simulink model "T3_updatesolarpart"  (R2022b)
settings: Solver=VariableStepAuto  StartTime=0.0  StopTime=10.0  RelTol=1e-3
undefined symbols (not defined in the file): High, Low
libraries: fl_lib x101, nesl_utility x52, simulink x14, ee_lib x5, slpidlib x2, eePwmGenerator x1
(part 3 of 3)

== system T3_updatesolarpart/Solar power/V ==
  PS-Simulink Converter : nesl_utility/PS-Simulink Converter  PhysicalDomain=network_engine_domain  SubClassName=ps_output  LeftPortType=input  RightPortType=output  PseudoPeriodic=off  Frequencies=[]  VectorFormat=inherit  Unit=inherit  AffineConversion=off
  Voltage Sensor : fl_lib/Electrical/Electrical Sensors/Voltage Sensor
  + : PMIOPort  Side=Left
  - : PMIOPort  Port=2  Side=Right
  tag scope: Vs=global
  wires:
  PS-Simulink Converter/1 -> [Vs]
  connections:
  PS-Simulink Converter/LConn1 -- Voltage Sensor/RConn1
  Voltage Sensor/LConn1 -- +/RConn1
  Voltage Sensor/RConn2 -- -/RConn1

== system T3_updatesolarpart/Wind energy/Subsystem ==
  Wind speed : Inport
  MATLAB System : MATLABSystem  System=windturbine_pitch_control  turbine_Pinst=1e6  turbine_dynamicsTimeConstant=5  inertia_dynamicsTimeConstant=3  Ts=0.01  SimulateUsing=Code generation
      mask Type: windturbine_pitch_control
      mask Display:
      | disp('windturbine_pitch_control');
      | port_label('input',1,'P_mechanic');
      | port_label('output',1,'P');
  Scope : Scope  NumInputPorts=2
  Wind turbine : Subsystem  mask{C1=0.5, C2=116, C3=0.4, C4=0, C5=5, C6=21, theta=0, W=1.57, R=40}
      mask prompts: C1 "coefficients C1"; C2 "coefficients C2"; C3 "coefficients C3"; C4 "coefficients C4"; C5 "coefficients C5"; C6 "coefficients C6"; theta "pitch angle"; W "angular velocity of rotor"; R "Blade Radius"
      mask DialogControl Container4 Prompt: Cp power coefficient
      mask DialogControl Container3 Prompt: Blade parameter
  Acitve power : Outport
  wires:
  Wind speed/1 -> Wind turbine/1(Vw wind speed)
  MATLAB System/1 -> Acitve power/1, Scope/2  "electrical"
  Wind turbine/1(Wind power) -> Scope/1, MATLAB System/1  "mechanical"

== system T3_updatesolarpart/Solar power/Boost Converter/AC Current Sensor1 ==
  Current Sensor : fl_lib/Electrical/Electrical Sensors/Current Sensor
  PS-Simulink Converter : nesl_utility/PS-Simulink Converter  PhysicalDomain=network_engine_domain  SubClassName=ps_output  LeftPortType=input  RightPortType=output  PseudoPeriodic=off  Frequencies=[]  VectorFormat=1-D array  Unit=1  AffineConversion=off
  - : PMIOPort  Side=Left
  + : PMIOPort  Port=2  Side=Right
  tag scope: Iboost=global
  wires:
  PS-Simulink Converter/1 -> [Iboost]
  connections:
  Current Sensor/RConn1 -- PS-Simulink Converter/LConn1
  +/RConn1 -- Current Sensor/LConn1
  Current Sensor/RConn2 -- -/RConn1

== system T3_updatesolarpart/Wind energy/Subsystem/Wind turbine ==
  Vw wind speed : Inport
  Blade radius : Constant  Value=R
  Constant : Constant  Value=1.225
  Multiply : Gain  Gain=1/2
  Multiply1 : Gain  Gain=pi
  Product : Product  Inputs=4
  Square : Math  Operator=square
  Subsystem : Subsystem
      mask Display: disp('Vw^3');
  Subsystem1 : Subsystem
  Wind power : Outport
  wires:
  Multiply/1 -> Wind power/1
  Product/1 -> Multiply/1
  Constant/1 -> Product/1  "Air density"
  Blade radius/1 -> Square/1
  Square/1 -> Multiply1/1
  Multiply1/1 -> Product/2  "Area"
  Vw wind speed/1 -> Subsystem1/1(Vw), Subsystem/1(In1)
  Subsystem1/1(Cp) -> Product/4
  Subsystem/1(Out1) -> Product/3

== system T3_updatesolarpart/Wind energy/Subsystem/Wind turbine/Subsystem ==
  In1 : Inport
  Square1 : Math  Operator=pow
  power of 3 : Constant  Value=3
  Out1 : Outport
  wires:
  power of 3/1 -> Square1/2
  Square1/1 -> Out1/1
  In1/1 -> Square1/1

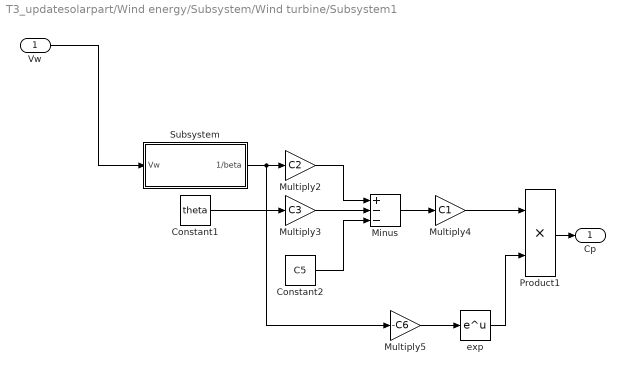
== system T3_updatesolarpart/Wind energy/Subsystem/Wind turbine/Subsystem1 ==
  Vw : Inport
  Constant1 : Constant  Value=theta
  Constant2 : Constant  Value=C5
  Minus : Sum  Inputs=+--
  Multiply2 : Gain  Gain=C2
  Multiply3 : Gain  Gain=C3
  Multiply4 : Gain  Gain=C1
  Multiply5 : Gain  Gain=-C6
  Product1 : Product
  Subsystem : Subsystem
  exp : Math
  Cp : Outport
  wires:
  Constant1/1 -> Multiply3/1
  Constant2/1 -> Minus/3
  Vw/1 -> Subsystem/1(Vw)
  Multiply2/1 -> Minus/1
  Minus/1 -> Multiply4/1
  Multiply4/1 -> Product1/1
  Subsystem/1(1/beta) -> Multiply5/1, Multiply2/1
  Multiply3/1 -> Minus/2
  exp/1 -> Product1/2
  Multiply5/1 -> exp/1
  Product1/1 -> Cp/1

== system T3_updatesolarpart/Wind energy/Subsystem/Wind turbine/Subsystem1/Subsystem ==
  Vw : Inport
  Constant : Constant  Value=theta
  MATLAB Function : MATLAB Function  TreatAsAtomicUnit=on
  Math Reciprocal : Math  Operator=reciprocal  SignedPower=on
  Multiply : Gain  Gain=R
  Multiply2 : Gain  Gain=W
  1/beta : Outport
  wires:
  Multiply/1 -> MATLAB Function/1(lambda)  "lambda"
  Constant/1 -> MATLAB Function/2(theta)
  MATLAB Function/1(beta) -> 1/beta/1  "1/beta"
  Vw/1 -> Math Reciprocal/1
  Multiply2/1 -> Multiply/1
  Math Reciprocal/1 -> Multiply2/1

== matlab function T3_updatesolarpart/Before t,off/MATLAB Function1 ==
  data: u input; y output; t input
function y = fcn(u,t)

y = -tanh(10000*(u-t))*1e6+1e6+1e-6;

== matlab function T3_updatesolarpart/Wind energy/Subsystem/Wind turbine/Subsystem1/Subsystem/MATLAB Function ==
  data: lambda input; beta output; theta input
function beta  = fcn(lambda,theta)
%#codegen
    beta= 1/(lambda+0.08*theta)-0.035/(1+theta^3);
end
